simulink model "comparator"  (R2018b)
settings: Solver=VariableStepAuto  StartTime=0.0  StopTime=10.0  RelTol=1e-3
libraries: simulink x1
settings Model: Creator=iamcy  LastModifiedBy=iamcy

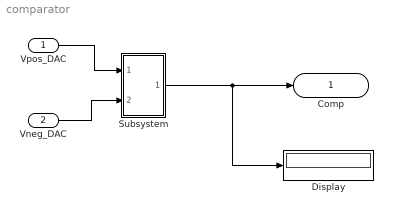
== system comparator ==
  Vpos_DAC : Inport
  Vneg_DAC : Inport  Port=2
  Display : Display
  Subsystem : Subsystem
  Comp : Outport  SignalName=Comp
  wires:
  Subsystem/1(Out1) -> Comp/1, Display/1
  Vpos_DAC/1 -> Subsystem/1(In1)
  Vneg_DAC/1 -> Subsystem/2(In2)

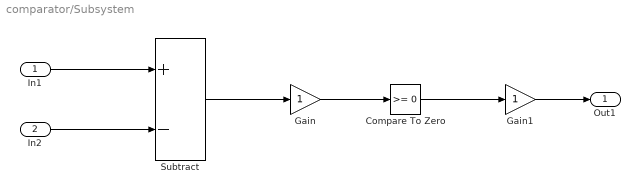
== system comparator/Subsystem ==
  In1 : Inport
  In2 : Inport  Port=2
  Compare To Zero : simulink/Logic and Bit Operations/Compare To Zero  relop=>=  OutDataTypeStr=boolean
  Gain : Gain
  Gain1 : Gain
  Subtract : Sum  Inputs=+-
  Out1 : Outport
  wires:
  Gain1/1 -> Out1/1
  Subtract/1 -> Gain/1
  Gain/1 -> Compare To Zero/1
  Compare To Zero/1 -> Gain1/1
  In2/1 -> Subtract/2
  In1/1 -> Subtract/1
